simulink model "ConsolidatedModelV0"  (R2022a)
settings: Solver=VariableStepAuto  StartTime=0.0  StopTime=10.0  RelTol=1e-3
libraries: commdigbbndpm3 x4, commblkcod2 x4, commchan3 x3, rllib x2, commsink2 x1
settings Model: Creator=yangz  LastModifiedBy=yangz

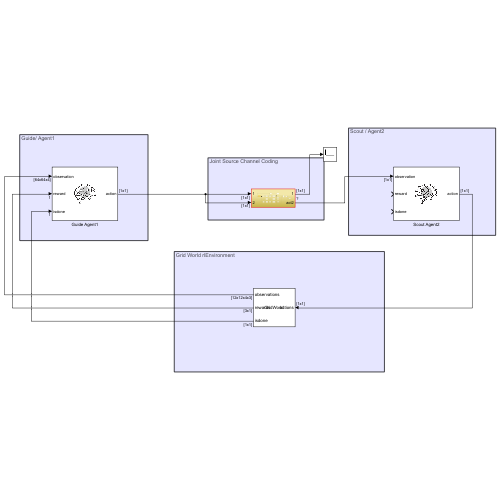
[thumbnail: Simulink's stored preview of the top-level diagram]
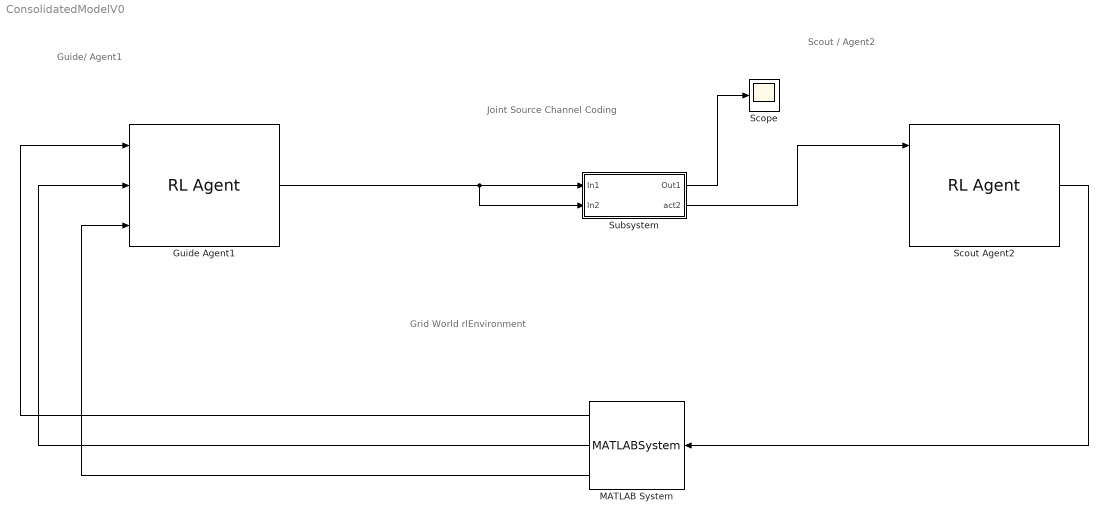
== system ConsolidatedModelV0 ==
  note: Joint Source Channel Coding
  note: Scout / Agent2
  note: Guide/ Agent1
  note: Grid World rlEnvironment
  Guide Agent1 : rllib/RL Agent  Agent=agent1  ExternalActionAsInput=off  ProvideLastAction=off  ProvideCumRwd=off  TreatAsDirectFeedthrough=on  UseStrictObservationDataTypes=off
  MATLAB System : MATLABSystem  System=GridWorld  InitialStates=[2 2;11 4;3 12]  Obstacles=-1  MaxStepCount=500  SimulateUsing=Code generation
      mask Type: GridWorld
      mask Display:
      | disp('GridWorld');
      | port_label('input',1,'actions');
      | port_label('output',1,'observations');
      | port_label('output',2,'rewards');
      | port_label('output',3,'isdone');
  Scope : Scope
  Scout Agent2 : rllib/RL Agent  Agent=agent2  ExternalActionAsInput=off  ProvideLastAction=off  ProvideCumRwd=off  TreatAsDirectFeedthrough=on  UseStrictObservationDataTypes=off
  Subsystem : Subsystem
  wires:
  Guide Agent1/1 -> Subsystem/2(In2), Subsystem/1(In1)
  Scout Agent2/1 -> MATLAB System/1
  MATLAB System/1 -> Guide Agent1/1
  MATLAB System/2 -> Guide Agent1/2
  MATLAB System/3 -> Guide Agent1/3
  Subsystem/2(act2) -> Scout Agent2/1
  Subsystem/1(Out1) -> Scope/1

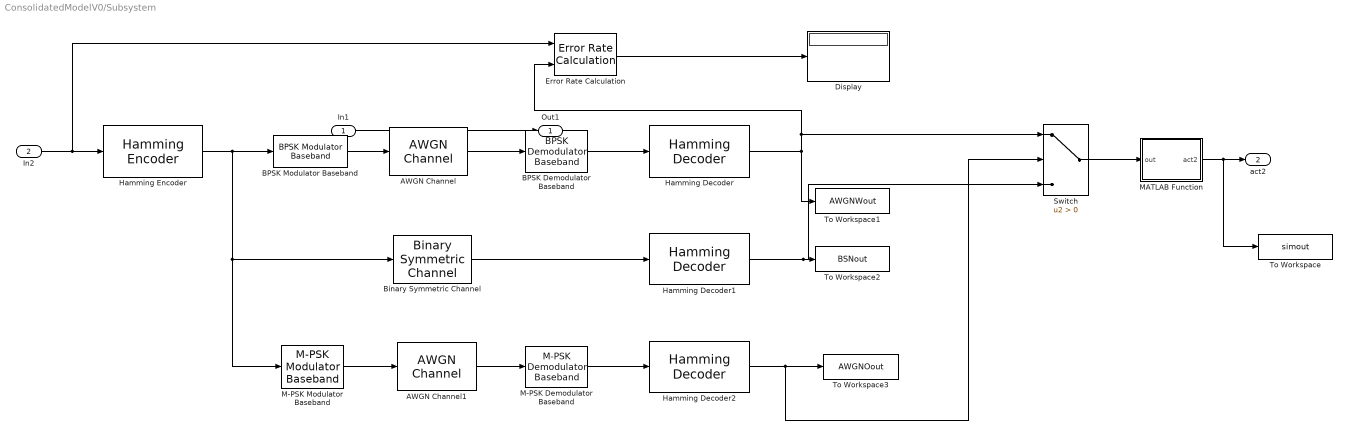
== system ConsolidatedModelV0/Subsystem ==
  In1 : Inport
  In2 : Inport  Port=2
  AWGN Channel : commchan3/AWGN Channel  InputProcessing=Columns as channels (frame based)  seed=67  noiseMode="Signal to noise ratio  (SNR)"  EbNodB=10  EsNodB=10  SNRdB=10  bitsPerSym=1  Ps=1  Tsym=1  variance=1
  AWGN Channel1 : commchan3/AWGN Channel  InputProcessing=Columns as channels (frame based)  seed=67  noiseMode="Signal to noise ratio  (SNR)"  EbNodB=10  EsNodB=10  SNRdB=10  bitsPerSym=1  Ps=1  Tsym=1  variance=1
  BPSK Demodulator Baseband : commdigbbndpm3/BPSK Demodulator Baseband  DecType=Hard decision  VarSource=Dialog  Variance=1  Ph=0  outDtype=Inherit via internal rule  derotateFactorWordLen=16  derotateFactorDataTypeStr=Inherit: Same word length as input  derotateFactorLastDataTypeStr=Inherit: Same word length as input
  BPSK Modulator Baseband : commdigbbndpm3/BPSK Modulator Baseband  Ph=0  outDtype=double  outWordLen=16  outUDDataType=sfix(16)  outFracLenMode=Best precision  outFracLen=15  outDataTypeStr=double  outLastDataTypeStr=double
  Binary Symmetric Channel : commchan3/Binary Symmetric Channel  ErrorProbability=0.05  ErrorVectorOutputPort=off  OutputDataType=double  OutputDataTypeSL=double  Seed=71  SimulateUsing=Code generation
      settings: SourceProductBaseCode=CM
  Display : Display
  Error Rate Calculation : commsink2/Error Rate Calculation  N=0  st_delay=0  cp_mode=Entire frame  subframe=[]  PMode=Port  WsName=ErrorVec  RsMode2=off  stop=off  numErr=100  maxBits=1e6
  Hamming Decoder : commblkcod2/Hamming Decoder  n=7  k=4
      settings: SourceProductBaseCode=CM
  Hamming Decoder1 : commblkcod2/Hamming Decoder  n=7  k=4
      settings: SourceProductBaseCode=CM
  Hamming Decoder2 : commblkcod2/Hamming Decoder  n=7  k=4
      settings: SourceProductBaseCode=CM
  Hamming Encoder : commblkcod2/Hamming Encoder  n=7  k=4
      settings: SourceProductBaseCode=CM
  M-PSK Demodulator Baseband : commdigbbndpm3/M-PSK Demodulator Baseband  M=8  OutType=Integer  DecType=Hard decision  VarSource=Dialog  Variance=1  Dec=Gray  Mapping=[0:7]  Ph=pi/8  outDtype1=Inherit via internal rule  outDtype2=Inherit via internal rule  derotateFactorWordLen=16  derotateFactorDataTypeStr=Inherit: Same word length as input  derotateFactorLastDataTypeStr=Inherit: Same word length as input
  M-PSK Modulator Baseband : commdigbbndpm3/M-PSK Modulator Baseband  M=8  InType=Integer  Enc=Gray  Mapping=[0:7]  Ph=pi/8  outDtype=double  outWordLen=16  outUDDataType=sfix(16)  outFracLenMode=Best precision  outFracLen=15  outDataTypeStr=double  outLastDataTypeStr=double
  MATLAB Function : MATLAB Function  TreatAsAtomicUnit=on
  Switch : Switch  Criteria=u2 > Threshold  SaturateOnIntegerOverflow=off  InputSameDT=off
  To Workspace : ToWorkspace  VariableName=simout  SaveFormat=Timeseries  SampleTime=-1
  To Workspace1 : ToWorkspace  VariableName=AWGNWout  SaveFormat=Timeseries  SampleTime=-1
  To Workspace2 : ToWorkspace  VariableName=BSNout  SaveFormat=Timeseries  SampleTime=-1
  To Workspace3 : ToWorkspace  VariableName=AWGNOout  SaveFormat=Timeseries  SampleTime=-1
  Out1 : Outport
  act2 : Outport  Port=2
  wires:
  In1/1 -> Out1/1
  Hamming Decoder/1 -> Error Rate Calculation/2, Switch/1, To Workspace1/1
  AWGN Channel1/1 -> M-PSK Demodulator Baseband/1
  Hamming Encoder/1 -> M-PSK Modulator Baseband/1, Binary Symmetric Channel/1, BPSK Modulator Baseband/1
  Binary Symmetric Channel/1 -> Hamming Decoder1/1
  Hamming Decoder1/1 -> Switch/3, To Workspace2/1
  Hamming Decoder2/1 -> Switch/2, To Workspace3/1
  M-PSK Demodulator Baseband/1 -> Hamming Decoder2/1
  In2/1 -> Error Rate Calculation/1, Hamming Encoder/1
  BPSK Modulator Baseband/1 -> AWGN Channel/1
  BPSK Demodulator Baseband/1 -> Hamming Decoder/1
  AWGN Channel/1 -> BPSK Demodulator Baseband/1
  Error Rate Calculation/1 -> Display/1
  M-PSK Modulator Baseband/1 -> AWGN Channel1/1
  Switch/1 -> MATLAB Function/1(out)
  MATLAB Function/1(act2) -> To Workspace/1, act2/1

== matlab function ConsolidatedModelV0/Subsystem/MATLAB Function ==
  data: out input; act2 output
function act2 = simouttodec(out)
lenData = length(out.simout2.Data);
for i = lenData
    for m = 1:4

elements(1:m,1:lenData) = out.simout.Data(1:m,1,1:lenData)
    end
end
trnEle = transpose(elements);
% % reshaped = reshape(vertcat(num2str(squeeze(elements))),size(1,elements),[])
 ele2str = num2str(elements);
 strTrnEle = num2str(trnEle)
 trnEle = transpose(ele2str);
% [GC GE] = groupcounts(trnFlat); % GC = "Element Occurances" GE = "Element Categories"
% % emptyCell = arrayfun(@isempty,trnFlat)
% % noEmptu =trnFlat(~emptyCell)n
% % noEmpty = arrayfun(@(x) x(~(x == "")),trnFlat)
 n = 1;
for i = 1: length(trnFlat)   
     if isempty(str2num(trnEle(i,:))) ~= 0
         noEmpty(n) = trnEle(i,:);       
          n = n+1;
     end
 
end 

% noEmpty = arrayfun('isempty',trnFlat)
for i = 1:length(strTrnEle)
oneRow(i) = {append(strTrnEle(i,1),strTrnEle(i,4),strTrnEle(i,7),strTrnEle(i,10))}
end

oneCol = bin2dec(oneRow);
[M F] = mode(oneCol,1);
act2 = M;
% [row col] = find(act2)
end
